simulink model "Sim_main"  (R2025a)
settings: Solver=FixedStepAuto  StartTime=0.0  StopTime=8760  FixedStep=1  RelTol=1e-3
values from neighbouring files (symbols this model uses):
  A = R * 2 * H    [LCOW_calculation.m]    (also in RUN_Simulink_POOL.m; RUN_Simulink_RandomSet.m; RUN_Simulink_SINGLE.m = 12.786871552)
  Cf = 36000    [RUN_Simulink_POOL.m]    (also in RUN_Simulink_RandomSet.m; RUN_Simulink_SINGLE.m)
  CutIn = 3    [RUN_Simulink_POOL.m]    (also in RUN_Simulink_RandomSet.m; RUN_Simulink_SINGLE.m)
  IP1 = (n/(n-1))*P1*( (P2/P1)^((n-1)/n) - 1)    (= 259255.992944)    [RUN_Simulink_POOL.m]    (also in RUN_Simulink_RandomSet.m; RUN_Simulink_SINGLE.m)
  J1 = 1.5 * As    [RUN_Simulink_POOL.m]    (also in RUN_Simulink_RandomSet.m; RUN_Simulink_SINGLE.m = 4.38)
  Limit_Tor = Tor_rq * 0.5    (= 2.3371585434)    [RUN_Simulink_POOL.m]    (also in RUN_Simulink_RandomSet.m; RUN_Simulink_SINGLE.m = 3.45899464424)
  N_PV = data.N_PV(i)    [LCOW_calculation.m]    (also in MOO_Qp_LCOW_CO2.m = optimvar("N_PV","Type","integer","LowerBound",1,"UpperBound"; RUN_Simulink_POOL.m = N_PV_values(i); RUN_Simulink_RandomSet.m = N_PV_values; RUN_Simulink_SINGLE.m = 2)
  N_ro = data.N_ro(i)    [LCOW_calculation.m]    (also in MOO_Qp_LCOW_CO2.m = optimvar("N_ro","Type","integer","LowerBound",2,"UpperBound"; RUN_Simulink_POOL.m = N_ro_values(i); RUN_Simulink_RandomSet.m = N_ro_values; RUN_Simulink_SINGLE.m = 6)
  Nt = data.Nt(i)    [LCOW_calculation.m]    (also in MOO_Qp_LCOW_CO2.m = optimvar("Nt","Type","integer","LowerBound",10,"UpperBound",; RUN_Simulink_POOL.m = Nt_values(i); RUN_Simulink_RandomSet.m = Nt_values; RUN_Simulink_SINGLE.m = 58)
  P2 = 800000    [RUN_Simulink_POOL.m]    (also in RUN_Simulink_RandomSet.m; RUN_Simulink_SINGLE.m)
  R = 0.515 * As    [LCOW_calculation.m]    (also in RUN_Simulink_POOL.m; RUN_Simulink_RandomSet.m; RUN_Simulink_SINGLE.m = 1.5038)
  Tor_rq = IP1 * Va * 10 / (17 * pi)    (= 4.67431708681)    [RUN_Simulink_POOL.m]    (also in RUN_Simulink_RandomSet.m; RUN_Simulink_SINGLE.m = 6.91798928848)
  TR = data.TR(i)    [LCOW_calculation.m]    (also in MOO_Qp_LCOW_CO2.m = optimvar("TR","LowerBound",3,"UpperBound",10); RUN_Simulink_POOL.m = TR_values(i); RUN_Simulink_RandomSet.m = TR_values; RUN_Simulink_SINGLE.m = 9.36)
  Va = e_vol * Vs    (= 9.6291546017e-05)    [RUN_Simulink_POOL.m]    (also in RUN_Simulink_RandomSet.m; RUN_Simulink_SINGLE.m = 0.000142511488105)
  Vf1 = ((P1+Pa)*T2/(T1*(P2+Pa)))*1000    (= 339.891157105)    [RUN_Simulink_POOL.m]    (also in RUN_Simulink_RandomSet.m; RUN_Simulink_SINGLE.m)
  Vt = 2000    [RUN_Simulink_POOL.m]    (also in RUN_Simulink_RandomSet.m; RUN_Simulink_SINGLE.m)
undefined symbols (not defined in the file or in its folder): magnitude
libraries: statsLibrary x36, simulink x1
(part 4 of 4)

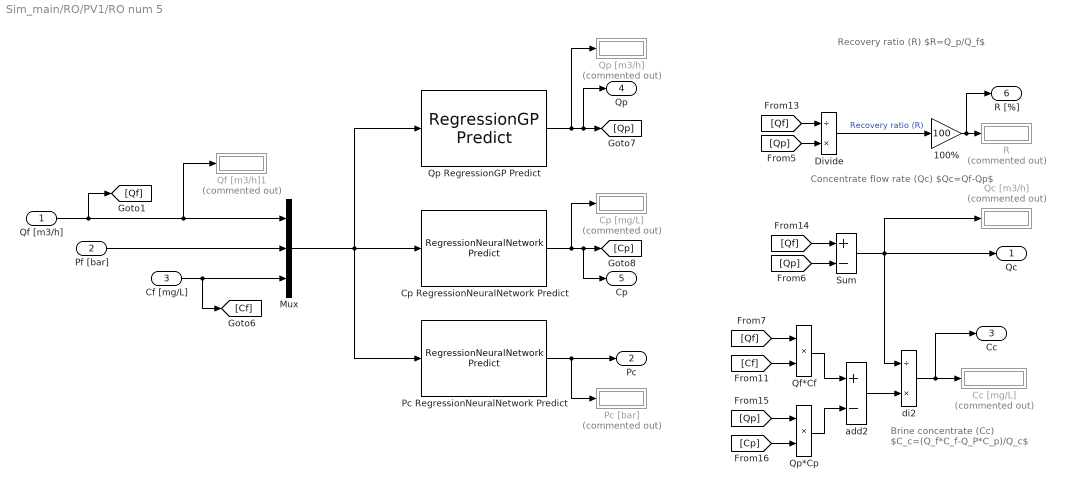
== system Sim_main/RO/PV1/RO num 5 ==
  note: Recovery ratio (R)
      | $R=Q_p/Q_f$
  note: Concentrate flow rate (Qc)
      | $Qc=Qf-Qp$
  note: Brine concentrate (Cc)
      | $C_c=(Q_f*C_f-Q_P*C_p)/Q_c$
  Qf [m3/h] : Inport
  Pf [bar] : Inport  Port=2
  Cf [mg/L] : Inport  Port=3
  100% : Gain  Gain=100
  Cc [mg/L] : Display  Commented=on
      settings: Format=bank
  Cp RegressionNeuralNetwork Predict : statsLibrary/Regression/RegressionNeuralNetwork Predict  TrainedLearner=RO_Cp.RegressionNeuralNetwork  OutMin=[]  OutMax=[]  OutputLayerOutMin=[]  OutputLayerOutMax=[]  OutputLayerAdditionOutMin=[]  OutputLayerAdditionOutMax=[]  LayerSelector=Layer 1  Layer1OutMin=[]  Layer1OutMax=[]  Layer1AdditionOutMin=[]  Layer1AdditionOutMax=[]  Layer2OutMin=[]  Layer2OutMax=[]  Layer2AdditionOutMin=[]  Layer2AdditionOutMax=[]  Layer3OutMin=[]  Layer3OutMax=[]  Layer3AdditionOutMin=[]  Layer3AdditionOutMax=[]  Layer4OutMin=[]  Layer4OutMax=[]  Layer4AdditionOutMin=[]  Layer4AdditionOutMax=[]  Layer5OutMin=[]  Layer5OutMax=[]  Layer5AdditionOutMin=[]  Layer5AdditionOutMax=[]  Layer6OutMin=[]  Layer6OutMax=[]  Layer6AdditionOutMin=[]  Layer6AdditionOutMax=[]  Layer7OutMin=[]  Layer7OutMax=[]  Layer7AdditionOutMin=[]  Layer7AdditionOutMax=[]  Layer8OutMin=[]  Layer8OutMax=[]  Layer8AdditionOutMin=[]  Layer8AdditionOutMax=[]  Layer9OutMin=[]  Layer9OutMax=[]  Layer9AdditionOutMin=[]  Layer9AdditionOutMax=[]  Layer10OutMin=[]  Layer10OutMax=[]  Layer10AdditionOutMin=[]  Layer10AdditionOutMax=[]  Layer11OutMin=[]  Layer11OutMax=[]  Layer11AdditionOutMin=[]  Layer11AdditionOutMax=[]  StandardizedInputOutMin=[]  StandardizedInputOutMax=[]  NumHiddenLayers=1
  Cp [mg/L] : Display  Commented=on
  Divide : Product  Inputs=/*
  Mux : Mux  Inputs=3
  Pc RegressionNeuralNetwork Predict : statsLibrary/Regression/RegressionNeuralNetwork Predict  TrainedLearner=RO_Pc.RegressionNeuralNetwork  OutMin=[]  OutMax=[]  OutputLayerOutMin=[]  OutputLayerOutMax=[]  OutputLayerAdditionOutMin=[]  OutputLayerAdditionOutMax=[]  LayerSelector=Layer 1  Layer1OutMin=[]  Layer1OutMax=[]  Layer1AdditionOutMin=[]  Layer1AdditionOutMax=[]  Layer2OutMin=[]  Layer2OutMax=[]  Layer2AdditionOutMin=[]  Layer2AdditionOutMax=[]  Layer3OutMin=[]  Layer3OutMax=[]  Layer3AdditionOutMin=[]  Layer3AdditionOutMax=[]  Layer4OutMin=[]  Layer4OutMax=[]  Layer4AdditionOutMin=[]  Layer4AdditionOutMax=[]  Layer5OutMin=[]  Layer5OutMax=[]  Layer5AdditionOutMin=[]  Layer5AdditionOutMax=[]  Layer6OutMin=[]  Layer6OutMax=[]  Layer6AdditionOutMin=[]  Layer6AdditionOutMax=[]  Layer7OutMin=[]  Layer7OutMax=[]  Layer7AdditionOutMin=[]  Layer7AdditionOutMax=[]  Layer8OutMin=[]  Layer8OutMax=[]  Layer8AdditionOutMin=[]  Layer8AdditionOutMax=[]  Layer9OutMin=[]  Layer9OutMax=[]  Layer9AdditionOutMin=[]  Layer9AdditionOutMax=[]  Layer10OutMin=[]  Layer10OutMax=[]  Layer10AdditionOutMin=[]  Layer10AdditionOutMax=[]  Layer11OutMin=[]  Layer11OutMax=[]  Layer11AdditionOutMin=[]  Layer11AdditionOutMax=[]  StandardizedInputOutMin=[]  StandardizedInputOutMax=[]  NumHiddenLayers=1
  Pc [bar] : Display  Commented=on
  Qc [m3/h] : Display  Commented=on
  Qf [m3/h]1 : Display  Commented=on
  Qf*Cf : Product
  Qp RegressionGP Predict : statsLibrary/Regression/RegressionGP Predict  TrainedLearner=RO_Qp.RegressionGP  ShowOutputSD=off  ShowOutputIntervals=off  Alpha=0.05  OutMin=[]  OutMax=[]  SDOutMin=[]  SDOutMax=[]  IntervalsOutMin=[]  IntervalsOutMax=[]  KernelMin=[]  KernelMax=[]  DistanceOutMin=[]  DistanceOutMax=[]  BasisOutMin=[]  BasisOutMax=[]  StandardizedInputOutMin=[]  StandardizedInputOutMax=[]  KernelParam1Min=[]  KernelParam1Max=[]  KernelParam2Min=[]  KernelParam2Max=[]  KernelParam3Min=[]  KernelParam3Max=[]  KernelParam4Min=[]  KernelParam4Max=[]  BasisParam1Min=[]  BasisParam1Max=[]  BasisParam2Min=[]  BasisParam2Max=[]  SDParam1Min=[]  SDParam1Max=[]  KernelParam5Min=[]  KernelParam5Max=[]
  Qp [m3/h] : Display  Commented=on
  Qp*Cp : Product
  R : Display  Commented=on
  Sum : Sum  Inputs=+-
  add2 : Sum  Inputs=+-
  di2 : Product  Inputs=/*
  Qc : Outport
  Pc : Outport  Port=2
  Cc : Outport  Port=3
  Qp : Outport  Port=4
  Cp : Outport  Port=5
  R [%] : Outport  Port=6
  wires:
  Cp RegressionNeuralNetwork Predict/1 -> Cp/1, [Cp], Cp [mg/L]/1
  Pc RegressionNeuralNetwork Predict/1 -> Pc/1, Pc [bar]/1
  Divide/1 -> 100%/1  "Recovery ratio (R)"
  Cf [mg/L]/1 -> Mux/3, [Cf]
  Mux/1 -> Pc RegressionNeuralNetwork Predict/1, Qp RegressionGP Predict/1, Cp RegressionNeuralNetwork Predict/1
  Pf [bar]/1 -> Mux/2
  Qf [m3/h]/1 -> [Qf], Qf [m3/h]1/1, Mux/1
  100%/1 -> R/1, R [%]/1
  Qp RegressionGP Predict/1 -> Qp/1, [Qp], Qp [m3/h]/1
  Sum/1 -> di2/1, Qc/1, Qc [m3/h]/1
  [Qf] -> Qf*Cf/1
  Qf*Cf/1 -> add2/1
  [Qp] -> Qp*Cp/1
  [Cf] -> Qf*Cf/2
  [Cp] -> Qp*Cp/2
  Qp*Cp/1 -> add2/2
  [Qf] -> Divide/1
  [Qp] -> Divide/2
  [Qf] -> Sum/1
  [Qp] -> Sum/2
  add2/1 -> di2/2
  di2/1 -> Cc/1, Cc [mg/L]/1

== system Sim_main/RO/PV1/RO num 6 ==
  note: Brine concentrate (Cc)
      | $C_c=(Q_f*C_f-Q_P*C_p)/Q_c$
  note: Concentrate flow rate (Qc)
      | $Qc=Qf-Qp$
  note: Recovery ratio (R)
      | $R=Q_p/Q_f$
  Qf [m3/h] : Inport
  Pf [bar] : Inport  Port=2
  Cf [mg/L] : Inport  Port=3
  100% : Gain  Gain=100
  Cc [mg/L] : Display  Commented=on
      settings: Format=bank
  Cp RegressionNeuralNetwork Predict : statsLibrary/Regression/RegressionNeuralNetwork Predict  TrainedLearner=RO_Cp.RegressionNeuralNetwork  OutMin=[]  OutMax=[]  OutputLayerOutMin=[]  OutputLayerOutMax=[]  OutputLayerAdditionOutMin=[]  OutputLayerAdditionOutMax=[]  LayerSelector=Layer 1  Layer1OutMin=[]  Layer1OutMax=[]  Layer1AdditionOutMin=[]  Layer1AdditionOutMax=[]  Layer2OutMin=[]  Layer2OutMax=[]  Layer2AdditionOutMin=[]  Layer2AdditionOutMax=[]  Layer3OutMin=[]  Layer3OutMax=[]  Layer3AdditionOutMin=[]  Layer3AdditionOutMax=[]  Layer4OutMin=[]  Layer4OutMax=[]  Layer4AdditionOutMin=[]  Layer4AdditionOutMax=[]  Layer5OutMin=[]  Layer5OutMax=[]  Layer5AdditionOutMin=[]  Layer5AdditionOutMax=[]  Layer6OutMin=[]  Layer6OutMax=[]  Layer6AdditionOutMin=[]  Layer6AdditionOutMax=[]  Layer7OutMin=[]  Layer7OutMax=[]  Layer7AdditionOutMin=[]  Layer7AdditionOutMax=[]  Layer8OutMin=[]  Layer8OutMax=[]  Layer8AdditionOutMin=[]  Layer8AdditionOutMax=[]  Layer9OutMin=[]  Layer9OutMax=[]  Layer9AdditionOutMin=[]  Layer9AdditionOutMax=[]  Layer10OutMin=[]  Layer10OutMax=[]  Layer10AdditionOutMin=[]  Layer10AdditionOutMax=[]  Layer11OutMin=[]  Layer11OutMax=[]  Layer11AdditionOutMin=[]  Layer11AdditionOutMax=[]  StandardizedInputOutMin=[]  StandardizedInputOutMax=[]  NumHiddenLayers=1
  Cp [mg/L] : Display  Commented=on
  Divide : Product  Inputs=/*
  Mux : Mux  Inputs=3
  Pc RegressionNeuralNetwork Predict : statsLibrary/Regression/RegressionNeuralNetwork Predict  TrainedLearner=RO_Pc.RegressionNeuralNetwork  OutMin=[]  OutMax=[]  OutputLayerOutMin=[]  OutputLayerOutMax=[]  OutputLayerAdditionOutMin=[]  OutputLayerAdditionOutMax=[]  LayerSelector=Layer 1  Layer1OutMin=[]  Layer1OutMax=[]  Layer1AdditionOutMin=[]  Layer1AdditionOutMax=[]  Layer2OutMin=[]  Layer2OutMax=[]  Layer2AdditionOutMin=[]  Layer2AdditionOutMax=[]  Layer3OutMin=[]  Layer3OutMax=[]  Layer3AdditionOutMin=[]  Layer3AdditionOutMax=[]  Layer4OutMin=[]  Layer4OutMax=[]  Layer4AdditionOutMin=[]  Layer4AdditionOutMax=[]  Layer5OutMin=[]  Layer5OutMax=[]  Layer5AdditionOutMin=[]  Layer5AdditionOutMax=[]  Layer6OutMin=[]  Layer6OutMax=[]  Layer6AdditionOutMin=[]  Layer6AdditionOutMax=[]  Layer7OutMin=[]  Layer7OutMax=[]  Layer7AdditionOutMin=[]  Layer7AdditionOutMax=[]  Layer8OutMin=[]  Layer8OutMax=[]  Layer8AdditionOutMin=[]  Layer8AdditionOutMax=[]  Layer9OutMin=[]  Layer9OutMax=[]  Layer9AdditionOutMin=[]  Layer9AdditionOutMax=[]  Layer10OutMin=[]  Layer10OutMax=[]  Layer10AdditionOutMin=[]  Layer10AdditionOutMax=[]  Layer11OutMin=[]  Layer11OutMax=[]  Layer11AdditionOutMin=[]  Layer11AdditionOutMax=[]  StandardizedInputOutMin=[]  StandardizedInputOutMax=[]  NumHiddenLayers=1
  Pc [bar] : Display  Commented=on
  Qc [m3/h] : Display  Commented=on
  Qf*Cf : Product
  Qp RegressionGP Predict : statsLibrary/Regression/RegressionGP Predict  TrainedLearner=RO_Qp.RegressionGP  ShowOutputSD=off  ShowOutputIntervals=off  Alpha=0.05  OutMin=[]  OutMax=[]  SDOutMin=[]  SDOutMax=[]  IntervalsOutMin=[]  IntervalsOutMax=[]  KernelMin=[]  KernelMax=[]  DistanceOutMin=[]  DistanceOutMax=[]  BasisOutMin=[]  BasisOutMax=[]  StandardizedInputOutMin=[]  StandardizedInputOutMax=[]  KernelParam1Min=[]  KernelParam1Max=[]  KernelParam2Min=[]  KernelParam2Max=[]  KernelParam3Min=[]  KernelParam3Max=[]  KernelParam4Min=[]  KernelParam4Max=[]  BasisParam1Min=[]  BasisParam1Max=[]  BasisParam2Min=[]  BasisParam2Max=[]  SDParam1Min=[]  SDParam1Max=[]  KernelParam5Min=[]  KernelParam5Max=[]
  Qp [m3/h] : Display  Commented=on
  Qp*Cp : Product
  R : Display  Commented=on
  Sum : Sum  Inputs=+-
  add2 : Sum  Inputs=+-
  di2 : Product  Inputs=/*
  Qc : Outport
  Pc : Outport  Port=2
  Cc : Outport  Port=3
  Qp : Outport  Port=4
  Cp : Outport  Port=5
  R [%] : Outport  Port=6
  wires:
  di2/1 -> Cc [mg/L]/1, Cc/1
  add2/1 -> di2/2
  [Qp] -> Sum/2
  [Qf] -> Sum/1
  [Qp] -> Divide/2
  [Qf] -> Divide/1
  Qp*Cp/1 -> add2/2
  [Cp] -> Qp*Cp/2
  [Cf] -> Qf*Cf/2
  [Qp] -> Qp*Cp/1
  Qf*Cf/1 -> add2/1
  [Qf] -> Qf*Cf/1
  Sum/1 -> Qc [m3/h]/1, Qc/1, di2/1
  Qp RegressionGP Predict/1 -> Qp [m3/h]/1, [Qp], Qp/1
  100%/1 -> R [%]/1, R/1
  Qf [m3/h]/1 -> Mux/1, [Qf]
  Pf [bar]/1 -> Mux/2
  Mux/1 -> Cp RegressionNeuralNetwork Predict/1, Qp RegressionGP Predict/1, Pc RegressionNeuralNetwork Predict/1
  Cf [mg/L]/1 -> [Cf], Mux/3
  Divide/1 -> 100%/1  "Recovery ratio (R)"
  Pc RegressionNeuralNetwork Predict/1 -> Pc [bar]/1, Pc/1
  Cp RegressionNeuralNetwork Predict/1 -> Cp [mg/L]/1, [Cp], Cp/1

== system Sim_main/RO/PV1/Subsystem ==
  note: product concentrate (Cp)
      | $C_3=(Q_1*C_1+Q_2*C_2)/Q_3$
  In1 : Inport
  In2 : Inport  Port=2
  In3 : Inport  Port=3
  In4 : Inport  Port=4
  Add1 : Sum
  Q1*C1 : Product
  Q2*C2 : Product
  add2 : Sum
  di2 : Product  Inputs=/*
  Out1 : Outport
  Out2 : Outport  Port=2
  wires:
  add2/1 -> di2/2
  In1/1 -> Add1/1, Q1*C1/1
  di2/1 -> Out1/1
  In3/1 -> Add1/2, Q2*C2/1
  Q1*C1/1 -> add2/1
  Q2*C2/1 -> add2/2
  Add1/1 -> di2/1, Out2/1
  In2/1 -> Q1*C1/2
  In4/1 -> Q2*C2/2

== system Sim_main/RO/PV1/Subsystem1 ==
  note: product concentrate (Cp)
      | $C_3=(Q_1*C_1+Q_2*C_2)/Q_3$
  In2 : Inport
  In3 : Inport  Port=2
  In4 : Inport  Port=3
  In1 : Inport  Port=4
  Add2 : Sum
  Q1*C1 : Product
  Q2*C2 : Product
  add2 : Sum
  di2 : Product  Inputs=/*
  Out1 : Outport
  Out2 : Outport  Port=2
  wires:
  di2/1 -> Out1/1
  add2/1 -> di2/2
  Q1*C1/1 -> add2/1
  Add2/1 -> di2/1, Out2/1
  In3/1 -> Q2*C2/1, Add2/2
  In4/1 -> Q2*C2/2
  Q2*C2/1 -> add2/2
  In2/1 -> Add2/1, Q1*C1/2
  In1/1 -> Q1*C1/1

== system Sim_main/RO/PV1/Subsystem2 ==
  note: product concentrate (Cp)
      | $C_3=(Q_1*C_1+Q_2*C_2)/Q_3$
  In2 : Inport
  In3 : Inport  Port=2
  In4 : Inport  Port=3
  In1 : Inport  Port=4
  Add2 : Sum
  Q1*C1 : Product
  Q2*C2 : Product
  add2 : Sum
  di2 : Product  Inputs=/*
  Out1 : Outport
  Out2 : Outport  Port=2
  wires:
  In1/1 -> Q1*C1/1
  In2/1 -> Q1*C1/2, Add2/1
  Q2*C2/1 -> add2/2
  In4/1 -> Q2*C2/2
  In3/1 -> Add2/2, Q2*C2/1
  Add2/1 -> Out2/1, di2/1
  Q1*C1/1 -> add2/1
  add2/1 -> di2/2
  di2/1 -> Out1/1

== system Sim_main/RO/PV1/Subsystem3 ==
  note: product concentrate (Cp)
      | $C_3=(Q_1*C_1+Q_2*C_2)/Q_3$
  In2 : Inport
  In3 : Inport  Port=2
  In4 : Inport  Port=3
  In1 : Inport  Port=4
  Add2 : Sum
  Q1*C1 : Product
  Q2*C2 : Product
  add2 : Sum
  di2 : Product  Inputs=/*
  Out1 : Outport
  wires:
  di2/1 -> Out1/1
  add2/1 -> di2/2
  Q1*C1/1 -> add2/1
  Add2/1 -> di2/1
  In3/1 -> Q2*C2/1, Add2/2
  In4/1 -> Q2*C2/2
  Q2*C2/1 -> add2/2
  In2/1 -> Add2/1, Q1*C1/2
  In1/1 -> Q1*C1/1

== system Sim_main/RO/PV1/Subsystem5 ==
  note: product concentrate (Cp)
      | $C_3=(Q_1*C_1+Q_2*C_2)/Q_3$
  In2 : Inport
  In3 : Inport  Port=2
  In4 : Inport  Port=3
  In1 : Inport  Port=4
  Add2 : Sum
  Q1*C1 : Product
  Q2*C2 : Product
  add2 : Sum
  di2 : Product  Inputs=/*
  Out1 : Outport
  Out2 : Outport  Port=2
  wires:
  In1/1 -> Q1*C1/1
  In2/1 -> Q1*C1/2, Add2/1
  Q2*C2/1 -> add2/2
  In4/1 -> Q2*C2/2
  In3/1 -> Add2/2, Q2*C2/1
  Add2/1 -> Out2/1, di2/1
  Q1*C1/1 -> add2/1
  add2/1 -> di2/2
  di2/1 -> Out1/1

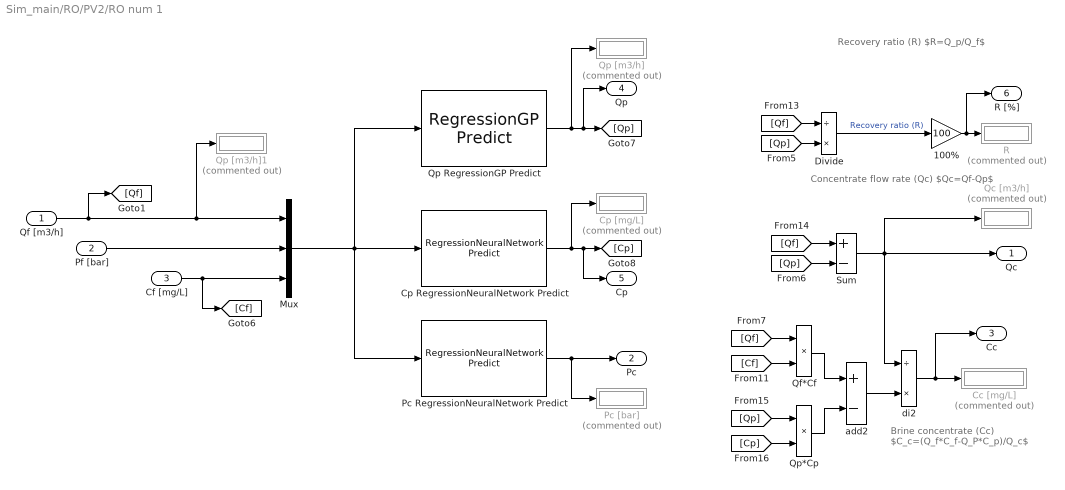
== system Sim_main/RO/PV2/RO num 1 ==
  note: Recovery ratio (R)
      | $R=Q_p/Q_f$
  note: Concentrate flow rate (Qc)
      | $Qc=Qf-Qp$
  note: Brine concentrate (Cc)
      | $C_c=(Q_f*C_f-Q_P*C_p)/Q_c$
  Qf [m3/h] : Inport
  Pf [bar] : Inport  Port=2
  Cf [mg/L] : Inport  Port=3
  100% : Gain  Gain=100
  Cc [mg/L] : Display  Commented=on
      settings: Format=bank
  Cp RegressionNeuralNetwork Predict : statsLibrary/Regression/RegressionNeuralNetwork Predict  TrainedLearner=RO_Cp.RegressionNeuralNetwork  OutMin=[]  OutMax=[]  OutputLayerOutMin=[]  OutputLayerOutMax=[]  OutputLayerAdditionOutMin=[]  OutputLayerAdditionOutMax=[]  LayerSelector=Layer 1  Layer1OutMin=[]  Layer1OutMax=[]  Layer1AdditionOutMin=[]  Layer1AdditionOutMax=[]  Layer2OutMin=[]  Layer2OutMax=[]  Layer2AdditionOutMin=[]  Layer2AdditionOutMax=[]  Layer3OutMin=[]  Layer3OutMax=[]  Layer3AdditionOutMin=[]  Layer3AdditionOutMax=[]  Layer4OutMin=[]  Layer4OutMax=[]  Layer4AdditionOutMin=[]  Layer4AdditionOutMax=[]  Layer5OutMin=[]  Layer5OutMax=[]  Layer5AdditionOutMin=[]  Layer5AdditionOutMax=[]  Layer6OutMin=[]  Layer6OutMax=[]  Layer6AdditionOutMin=[]  Layer6AdditionOutMax=[]  Layer7OutMin=[]  Layer7OutMax=[]  Layer7AdditionOutMin=[]  Layer7AdditionOutMax=[]  Layer8OutMin=[]  Layer8OutMax=[]  Layer8AdditionOutMin=[]  Layer8AdditionOutMax=[]  Layer9OutMin=[]  Layer9OutMax=[]  Layer9AdditionOutMin=[]  Layer9AdditionOutMax=[]  Layer10OutMin=[]  Layer10OutMax=[]  Layer10AdditionOutMin=[]  Layer10AdditionOutMax=[]  Layer11OutMin=[]  Layer11OutMax=[]  Layer11AdditionOutMin=[]  Layer11AdditionOutMax=[]  StandardizedInputOutMin=[]  StandardizedInputOutMax=[]  NumHiddenLayers=1
  Cp [mg/L] : Display  Commented=on
  Divide : Product  Inputs=/*
  Mux : Mux  Inputs=3
  Pc RegressionNeuralNetwork Predict : statsLibrary/Regression/RegressionNeuralNetwork Predict  TrainedLearner=RO_Pc.RegressionNeuralNetwork  OutMin=[]  OutMax=[]  OutputLayerOutMin=[]  OutputLayerOutMax=[]  OutputLayerAdditionOutMin=[]  OutputLayerAdditionOutMax=[]  LayerSelector=Layer 1  Layer1OutMin=[]  Layer1OutMax=[]  Layer1AdditionOutMin=[]  Layer1AdditionOutMax=[]  Layer2OutMin=[]  Layer2OutMax=[]  Layer2AdditionOutMin=[]  Layer2AdditionOutMax=[]  Layer3OutMin=[]  Layer3OutMax=[]  Layer3AdditionOutMin=[]  Layer3AdditionOutMax=[]  Layer4OutMin=[]  Layer4OutMax=[]  Layer4AdditionOutMin=[]  Layer4AdditionOutMax=[]  Layer5OutMin=[]  Layer5OutMax=[]  Layer5AdditionOutMin=[]  Layer5AdditionOutMax=[]  Layer6OutMin=[]  Layer6OutMax=[]  Layer6AdditionOutMin=[]  Layer6AdditionOutMax=[]  Layer7OutMin=[]  Layer7OutMax=[]  Layer7AdditionOutMin=[]  Layer7AdditionOutMax=[]  Layer8OutMin=[]  Layer8OutMax=[]  Layer8AdditionOutMin=[]  Layer8AdditionOutMax=[]  Layer9OutMin=[]  Layer9OutMax=[]  Layer9AdditionOutMin=[]  Layer9AdditionOutMax=[]  Layer10OutMin=[]  Layer10OutMax=[]  Layer10AdditionOutMin=[]  Layer10AdditionOutMax=[]  Layer11OutMin=[]  Layer11OutMax=[]  Layer11AdditionOutMin=[]  Layer11AdditionOutMax=[]  StandardizedInputOutMin=[]  StandardizedInputOutMax=[]  NumHiddenLayers=1
  Pc [bar] : Display  Commented=on
  Qc [m3/h] : Display  Commented=on
  Qf*Cf : Product
  Qp RegressionGP Predict : statsLibrary/Regression/RegressionGP Predict  TrainedLearner=RO_Qp.RegressionGP  ShowOutputSD=off  ShowOutputIntervals=off  Alpha=0.05  OutMin=[]  OutMax=[]  SDOutMin=[]  SDOutMax=[]  IntervalsOutMin=[]  IntervalsOutMax=[]  KernelMin=[]  KernelMax=[]  DistanceOutMin=[]  DistanceOutMax=[]  BasisOutMin=[]  BasisOutMax=[]  StandardizedInputOutMin=[]  StandardizedInputOutMax=[]  KernelParam1Min=[]  KernelParam1Max=[]  KernelParam2Min=[]  KernelParam2Max=[]  KernelParam3Min=[]  KernelParam3Max=[]  KernelParam4Min=[]  KernelParam4Max=[]  BasisParam1Min=[]  BasisParam1Max=[]  BasisParam2Min=[]  BasisParam2Max=[]  SDParam1Min=[]  SDParam1Max=[]  KernelParam5Min=[]  KernelParam5Max=[]
  Qp [m3/h] : Display  Commented=on
  Qp [m3/h]1 : Display  Commented=on
  Qp*Cp : Product
  R : Display  Commented=on
  Sum : Sum  Inputs=+-
  add2 : Sum  Inputs=+-
  di2 : Product  Inputs=/*
  Qc : Outport
  Pc : Outport  Port=2
  Cc : Outport  Port=3
  Qp : Outport  Port=4
  Cp : Outport  Port=5
  R [%] : Outport  Port=6
  wires:
  Cp RegressionNeuralNetwork Predict/1 -> Cp/1, [Cp], Cp [mg/L]/1
  Pc RegressionNeuralNetwork Predict/1 -> Pc/1, Pc [bar]/1
  Divide/1 -> 100%/1  "Recovery ratio (R)"
  Cf [mg/L]/1 -> Mux/3, [Cf]
  Mux/1 -> Pc RegressionNeuralNetwork Predict/1, Qp RegressionGP Predict/1, Cp RegressionNeuralNetwork Predict/1
  Pf [bar]/1 -> Mux/2
  100%/1 -> R/1, R [%]/1
  Qp RegressionGP Predict/1 -> Qp/1, [Qp], Qp [m3/h]/1
  Sum/1 -> di2/1, Qc/1, Qc [m3/h]/1
  [Qf] -> Qf*Cf/1
  Qf*Cf/1 -> add2/1
  [Qp] -> Qp*Cp/1
  [Cf] -> Qf*Cf/2
  [Cp] -> Qp*Cp/2
  Qp*Cp/1 -> add2/2
  [Qf] -> Divide/1
  [Qp] -> Divide/2
  [Qf] -> Sum/1
  [Qp] -> Sum/2
  add2/1 -> di2/2
  di2/1 -> Cc/1, Cc [mg/L]/1
  Qf [m3/h]/1 -> [Qf], Mux/1, Qp [m3/h]1/1

== system Sim_main/RO/PV2/RO num 2 ==
  note: Brine concentrate (Cc)
      | $C_c=(Q_f*C_f-Q_P*C_p)/Q_c$
  note: Concentrate flow rate (Qc)
      | $Qc=Qf-Qp$
  note: Recovery ratio (R)
      | $R=Q_p/Q_f$
  Qf [m3/h] : Inport
  Pf [bar] : Inport  Port=2
  Cf [mg/L] : Inport  Port=3
  100% : Gain  Gain=100
  Cc [mg/L] : Display  Commented=on
      settings: Format=bank
  Cp RegressionNeuralNetwork Predict : statsLibrary/Regression/RegressionNeuralNetwork Predict  TrainedLearner=RO_Cp.RegressionNeuralNetwork  OutMin=[]  OutMax=[]  OutputLayerOutMin=[]  OutputLayerOutMax=[]  OutputLayerAdditionOutMin=[]  OutputLayerAdditionOutMax=[]  LayerSelector=Layer 1  Layer1OutMin=[]  Layer1OutMax=[]  Layer1AdditionOutMin=[]  Layer1AdditionOutMax=[]  Layer2OutMin=[]  Layer2OutMax=[]  Layer2AdditionOutMin=[]  Layer2AdditionOutMax=[]  Layer3OutMin=[]  Layer3OutMax=[]  Layer3AdditionOutMin=[]  Layer3AdditionOutMax=[]  Layer4OutMin=[]  Layer4OutMax=[]  Layer4AdditionOutMin=[]  Layer4AdditionOutMax=[]  Layer5OutMin=[]  Layer5OutMax=[]  Layer5AdditionOutMin=[]  Layer5AdditionOutMax=[]  Layer6OutMin=[]  Layer6OutMax=[]  Layer6AdditionOutMin=[]  Layer6AdditionOutMax=[]  Layer7OutMin=[]  Layer7OutMax=[]  Layer7AdditionOutMin=[]  Layer7AdditionOutMax=[]  Layer8OutMin=[]  Layer8OutMax=[]  Layer8AdditionOutMin=[]  Layer8AdditionOutMax=[]  Layer9OutMin=[]  Layer9OutMax=[]  Layer9AdditionOutMin=[]  Layer9AdditionOutMax=[]  Layer10OutMin=[]  Layer10OutMax=[]  Layer10AdditionOutMin=[]  Layer10AdditionOutMax=[]  Layer11OutMin=[]  Layer11OutMax=[]  Layer11AdditionOutMin=[]  Layer11AdditionOutMax=[]  StandardizedInputOutMin=[]  StandardizedInputOutMax=[]  NumHiddenLayers=1
  Cp [mg/L] : Display  Commented=on
  Divide : Product  Inputs=/*
  Mux : Mux  Inputs=3
  Pc RegressionNeuralNetwork Predict : statsLibrary/Regression/RegressionNeuralNetwork Predict  TrainedLearner=RO_Pc.RegressionNeuralNetwork  OutMin=[]  OutMax=[]  OutputLayerOutMin=[]  OutputLayerOutMax=[]  OutputLayerAdditionOutMin=[]  OutputLayerAdditionOutMax=[]  LayerSelector=Layer 1  Layer1OutMin=[]  Layer1OutMax=[]  Layer1AdditionOutMin=[]  Layer1AdditionOutMax=[]  Layer2OutMin=[]  Layer2OutMax=[]  Layer2AdditionOutMin=[]  Layer2AdditionOutMax=[]  Layer3OutMin=[]  Layer3OutMax=[]  Layer3AdditionOutMin=[]  Layer3AdditionOutMax=[]  Layer4OutMin=[]  Layer4OutMax=[]  Layer4AdditionOutMin=[]  Layer4AdditionOutMax=[]  Layer5OutMin=[]  Layer5OutMax=[]  Layer5AdditionOutMin=[]  Layer5AdditionOutMax=[]  Layer6OutMin=[]  Layer6OutMax=[]  Layer6AdditionOutMin=[]  Layer6AdditionOutMax=[]  Layer7OutMin=[]  Layer7OutMax=[]  Layer7AdditionOutMin=[]  Layer7AdditionOutMax=[]  Layer8OutMin=[]  Layer8OutMax=[]  Layer8AdditionOutMin=[]  Layer8AdditionOutMax=[]  Layer9OutMin=[]  Layer9OutMax=[]  Layer9AdditionOutMin=[]  Layer9AdditionOutMax=[]  Layer10OutMin=[]  Layer10OutMax=[]  Layer10AdditionOutMin=[]  Layer10AdditionOutMax=[]  Layer11OutMin=[]  Layer11OutMax=[]  Layer11AdditionOutMin=[]  Layer11AdditionOutMax=[]  StandardizedInputOutMin=[]  StandardizedInputOutMax=[]  NumHiddenLayers=1
  Pc [bar] : Display  Commented=on
  Qc [m3/h] : Display  Commented=on
  Qf*Cf : Product
  Qp RegressionGP Predict : statsLibrary/Regression/RegressionGP Predict  TrainedLearner=RO_Qp.RegressionGP  ShowOutputSD=off  ShowOutputIntervals=off  Alpha=0.05  OutMin=[]  OutMax=[]  SDOutMin=[]  SDOutMax=[]  IntervalsOutMin=[]  IntervalsOutMax=[]  KernelMin=[]  KernelMax=[]  DistanceOutMin=[]  DistanceOutMax=[]  BasisOutMin=[]  BasisOutMax=[]  StandardizedInputOutMin=[]  StandardizedInputOutMax=[]  KernelParam1Min=[]  KernelParam1Max=[]  KernelParam2Min=[]  KernelParam2Max=[]  KernelParam3Min=[]  KernelParam3Max=[]  KernelParam4Min=[]  KernelParam4Max=[]  BasisParam1Min=[]  BasisParam1Max=[]  BasisParam2Min=[]  BasisParam2Max=[]  SDParam1Min=[]  SDParam1Max=[]  KernelParam5Min=[]  KernelParam5Max=[]
  Qp [m3/h] : Display  Commented=on
  Qp*Cp : Product
  R : Display  Commented=on
  Sum : Sum  Inputs=+-
  add2 : Sum  Inputs=+-
  di2 : Product  Inputs=/*
  Qc : Outport
  Pc : Outport  Port=2
  Cc : Outport  Port=3
  Qp : Outport  Port=4
  Cp : Outport  Port=5
  R [%] : Outport  Port=6
  wires:
  di2/1 -> Cc [mg/L]/1, Cc/1
  add2/1 -> di2/2
  [Qp] -> Sum/2
  [Qf] -> Sum/1
  [Qp] -> Divide/2
  [Qf] -> Divide/1
  Qp*Cp/1 -> add2/2
  [Cp] -> Qp*Cp/2
  [Cf] -> Qf*Cf/2
  [Qp] -> Qp*Cp/1
  Qf*Cf/1 -> add2/1
  [Qf] -> Qf*Cf/1
  Sum/1 -> Qc [m3/h]/1, Qc/1, di2/1
  Qp RegressionGP Predict/1 -> Qp [m3/h]/1, [Qp], Qp/1
  100%/1 -> R [%]/1, R/1
  Qf [m3/h]/1 -> Mux/1, [Qf]
  Pf [bar]/1 -> Mux/2
  Mux/1 -> Cp RegressionNeuralNetwork Predict/1, Qp RegressionGP Predict/1, Pc RegressionNeuralNetwork Predict/1
  Cf [mg/L]/1 -> [Cf], Mux/3
  Divide/1 -> 100%/1  "Recovery ratio (R)"
  Pc RegressionNeuralNetwork Predict/1 -> Pc [bar]/1, Pc/1
  Cp RegressionNeuralNetwork Predict/1 -> Cp [mg/L]/1, [Cp], Cp/1

== system Sim_main/RO/PV2/RO num 3 ==
  note: Recovery ratio (R)
      | $R=Q_p/Q_f$
  note: Concentrate flow rate (Qc)
      | $Qc=Qf-Qp$
  note: Brine concentrate (Cc)
      | $C_c=(Q_f*C_f-Q_P*C_p)/Q_c$
  Qf [m3/h] : Inport
  Pf [bar] : Inport  Port=2
  Cf [mg/L] : Inport  Port=3
  100% : Gain  Gain=100
  Cc [mg/L] : Display  Commented=on
      settings: Format=bank
  Cp RegressionNeuralNetwork Predict : statsLibrary/Regression/RegressionNeuralNetwork Predict  TrainedLearner=RO_Cp.RegressionNeuralNetwork  OutMin=[]  OutMax=[]  OutputLayerOutMin=[]  OutputLayerOutMax=[]  OutputLayerAdditionOutMin=[]  OutputLayerAdditionOutMax=[]  LayerSelector=Layer 1  Layer1OutMin=[]  Layer1OutMax=[]  Layer1AdditionOutMin=[]  Layer1AdditionOutMax=[]  Layer2OutMin=[]  Layer2OutMax=[]  Layer2AdditionOutMin=[]  Layer2AdditionOutMax=[]  Layer3OutMin=[]  Layer3OutMax=[]  Layer3AdditionOutMin=[]  Layer3AdditionOutMax=[]  Layer4OutMin=[]  Layer4OutMax=[]  Layer4AdditionOutMin=[]  Layer4AdditionOutMax=[]  Layer5OutMin=[]  Layer5OutMax=[]  Layer5AdditionOutMin=[]  Layer5AdditionOutMax=[]  Layer6OutMin=[]  Layer6OutMax=[]  Layer6AdditionOutMin=[]  Layer6AdditionOutMax=[]  Layer7OutMin=[]  Layer7OutMax=[]  Layer7AdditionOutMin=[]  Layer7AdditionOutMax=[]  Layer8OutMin=[]  Layer8OutMax=[]  Layer8AdditionOutMin=[]  Layer8AdditionOutMax=[]  Layer9OutMin=[]  Layer9OutMax=[]  Layer9AdditionOutMin=[]  Layer9AdditionOutMax=[]  Layer10OutMin=[]  Layer10OutMax=[]  Layer10AdditionOutMin=[]  Layer10AdditionOutMax=[]  Layer11OutMin=[]  Layer11OutMax=[]  Layer11AdditionOutMin=[]  Layer11AdditionOutMax=[]  StandardizedInputOutMin=[]  StandardizedInputOutMax=[]  NumHiddenLayers=1
  Cp [mg/L] : Display  Commented=on
  Divide : Product  Inputs=/*
  Mux : Mux  Inputs=3
  Pc RegressionNeuralNetwork Predict : statsLibrary/Regression/RegressionNeuralNetwork Predict  TrainedLearner=RO_Pc.RegressionNeuralNetwork  OutMin=[]  OutMax=[]  OutputLayerOutMin=[]  OutputLayerOutMax=[]  OutputLayerAdditionOutMin=[]  OutputLayerAdditionOutMax=[]  LayerSelector=Layer 1  Layer1OutMin=[]  Layer1OutMax=[]  Layer1AdditionOutMin=[]  Layer1AdditionOutMax=[]  Layer2OutMin=[]  Layer2OutMax=[]  Layer2AdditionOutMin=[]  Layer2AdditionOutMax=[]  Layer3OutMin=[]  Layer3OutMax=[]  Layer3AdditionOutMin=[]  Layer3AdditionOutMax=[]  Layer4OutMin=[]  Layer4OutMax=[]  Layer4AdditionOutMin=[]  Layer4AdditionOutMax=[]  Layer5OutMin=[]  Layer5OutMax=[]  Layer5AdditionOutMin=[]  Layer5AdditionOutMax=[]  Layer6OutMin=[]  Layer6OutMax=[]  Layer6AdditionOutMin=[]  Layer6AdditionOutMax=[]  Layer7OutMin=[]  Layer7OutMax=[]  Layer7AdditionOutMin=[]  Layer7AdditionOutMax=[]  Layer8OutMin=[]  Layer8OutMax=[]  Layer8AdditionOutMin=[]  Layer8AdditionOutMax=[]  Layer9OutMin=[]  Layer9OutMax=[]  Layer9AdditionOutMin=[]  Layer9AdditionOutMax=[]  Layer10OutMin=[]  Layer10OutMax=[]  Layer10AdditionOutMin=[]  Layer10AdditionOutMax=[]  Layer11OutMin=[]  Layer11OutMax=[]  Layer11AdditionOutMin=[]  Layer11AdditionOutMax=[]  StandardizedInputOutMin=[]  StandardizedInputOutMax=[]  NumHiddenLayers=1
  Pc [bar] : Display  Commented=on
  Qc [m3/h] : Display  Commented=on
  Qf*Cf : Product
  Qp RegressionGP Predict : statsLibrary/Regression/RegressionGP Predict  TrainedLearner=RO_Qp.RegressionGP  ShowOutputSD=off  ShowOutputIntervals=off  Alpha=0.05  OutMin=[]  OutMax=[]  SDOutMin=[]  SDOutMax=[]  IntervalsOutMin=[]  IntervalsOutMax=[]  KernelMin=[]  KernelMax=[]  DistanceOutMin=[]  DistanceOutMax=[]  BasisOutMin=[]  BasisOutMax=[]  StandardizedInputOutMin=[]  StandardizedInputOutMax=[]  KernelParam1Min=[]  KernelParam1Max=[]  KernelParam2Min=[]  KernelParam2Max=[]  KernelParam3Min=[]  KernelParam3Max=[]  KernelParam4Min=[]  KernelParam4Max=[]  BasisParam1Min=[]  BasisParam1Max=[]  BasisParam2Min=[]  BasisParam2Max=[]  SDParam1Min=[]  SDParam1Max=[]  KernelParam5Min=[]  KernelParam5Max=[]
  Qp [m3/h] : Display  Commented=on
  Qp*Cp : Product
  R : Display  Commented=on
  Sum : Sum  Inputs=+-
  add2 : Sum  Inputs=+-
  di2 : Product  Inputs=/*
  Qc : Outport
  Pc : Outport  Port=2
  Cc : Outport  Port=3
  Qp : Outport  Port=4
  Cp : Outport  Port=5
  R [%] : Outport  Port=6
  wires:
  Cp RegressionNeuralNetwork Predict/1 -> Cp/1, [Cp], Cp [mg/L]/1
  Pc RegressionNeuralNetwork Predict/1 -> Pc/1, Pc [bar]/1
  Divide/1 -> 100%/1  "Recovery ratio (R)"
  Cf [mg/L]/1 -> Mux/3, [Cf]
  Mux/1 -> Pc RegressionNeuralNetwork Predict/1, Qp RegressionGP Predict/1, Cp RegressionNeuralNetwork Predict/1
  Pf [bar]/1 -> Mux/2
  Qf [m3/h]/1 -> [Qf], Mux/1
  100%/1 -> R/1, R [%]/1
  Qp RegressionGP Predict/1 -> Qp/1, [Qp], Qp [m3/h]/1
  Sum/1 -> di2/1, Qc/1, Qc [m3/h]/1
  [Qf] -> Qf*Cf/1
  Qf*Cf/1 -> add2/1
  [Qp] -> Qp*Cp/1
  [Cf] -> Qf*Cf/2
  [Cp] -> Qp*Cp/2
  Qp*Cp/1 -> add2/2
  [Qf] -> Divide/1
  [Qp] -> Divide/2
  [Qf] -> Sum/1
  [Qp] -> Sum/2
  add2/1 -> di2/2
  di2/1 -> Cc/1, Cc [mg/L]/1

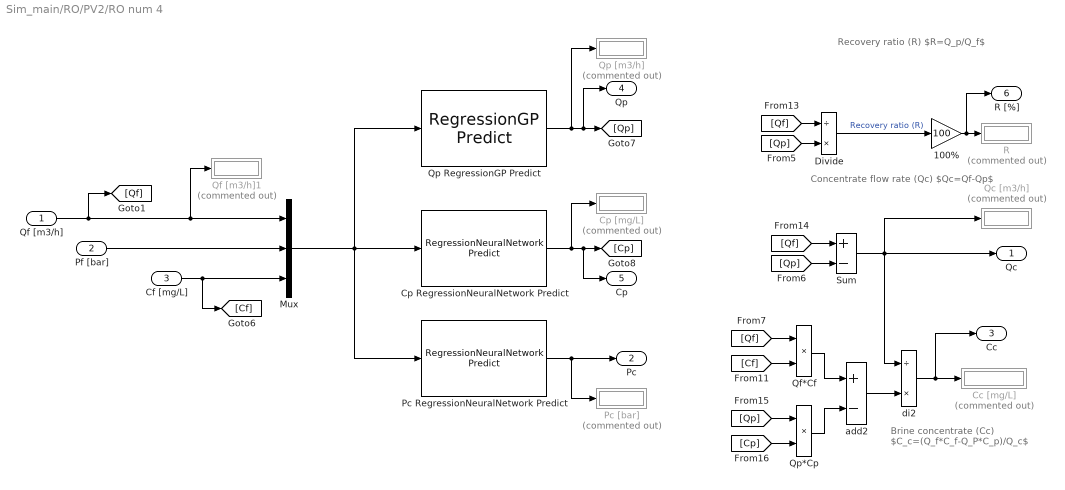
== system Sim_main/RO/PV2/RO num 4 ==
  note: Brine concentrate (Cc)
      | $C_c=(Q_f*C_f-Q_P*C_p)/Q_c$
  note: Concentrate flow rate (Qc)
      | $Qc=Qf-Qp$
  note: Recovery ratio (R)
      | $R=Q_p/Q_f$
  Qf [m3/h] : Inport
  Pf [bar] : Inport  Port=2
  Cf [mg/L] : Inport  Port=3
  100% : Gain  Gain=100
  Cc [mg/L] : Display  Commented=on
      settings: Format=bank
  Cp RegressionNeuralNetwork Predict : statsLibrary/Regression/RegressionNeuralNetwork Predict  TrainedLearner=RO_Cp.RegressionNeuralNetwork  OutMin=[]  OutMax=[]  OutputLayerOutMin=[]  OutputLayerOutMax=[]  OutputLayerAdditionOutMin=[]  OutputLayerAdditionOutMax=[]  LayerSelector=Layer 1  Layer1OutMin=[]  Layer1OutMax=[]  Layer1AdditionOutMin=[]  Layer1AdditionOutMax=[]  Layer2OutMin=[]  Layer2OutMax=[]  Layer2AdditionOutMin=[]  Layer2AdditionOutMax=[]  Layer3OutMin=[]  Layer3OutMax=[]  Layer3AdditionOutMin=[]  Layer3AdditionOutMax=[]  Layer4OutMin=[]  Layer4OutMax=[]  Layer4AdditionOutMin=[]  Layer4AdditionOutMax=[]  Layer5OutMin=[]  Layer5OutMax=[]  Layer5AdditionOutMin=[]  Layer5AdditionOutMax=[]  Layer6OutMin=[]  Layer6OutMax=[]  Layer6AdditionOutMin=[]  Layer6AdditionOutMax=[]  Layer7OutMin=[]  Layer7OutMax=[]  Layer7AdditionOutMin=[]  Layer7AdditionOutMax=[]  Layer8OutMin=[]  Layer8OutMax=[]  Layer8AdditionOutMin=[]  Layer8AdditionOutMax=[]  Layer9OutMin=[]  Layer9OutMax=[]  Layer9AdditionOutMin=[]  Layer9AdditionOutMax=[]  Layer10OutMin=[]  Layer10OutMax=[]  Layer10AdditionOutMin=[]  Layer10AdditionOutMax=[]  Layer11OutMin=[]  Layer11OutMax=[]  Layer11AdditionOutMin=[]  Layer11AdditionOutMax=[]  StandardizedInputOutMin=[]  StandardizedInputOutMax=[]  NumHiddenLayers=1
  Cp [mg/L] : Display  Commented=on
  Divide : Product  Inputs=/*
  Mux : Mux  Inputs=3
  Pc RegressionNeuralNetwork Predict : statsLibrary/Regression/RegressionNeuralNetwork Predict  TrainedLearner=RO_Pc.RegressionNeuralNetwork  OutMin=[]  OutMax=[]  OutputLayerOutMin=[]  OutputLayerOutMax=[]  OutputLayerAdditionOutMin=[]  OutputLayerAdditionOutMax=[]  LayerSelector=Layer 1  Layer1OutMin=[]  Layer1OutMax=[]  Layer1AdditionOutMin=[]  Layer1AdditionOutMax=[]  Layer2OutMin=[]  Layer2OutMax=[]  Layer2AdditionOutMin=[]  Layer2AdditionOutMax=[]  Layer3OutMin=[]  Layer3OutMax=[]  Layer3AdditionOutMin=[]  Layer3AdditionOutMax=[]  Layer4OutMin=[]  Layer4OutMax=[]  Layer4AdditionOutMin=[]  Layer4AdditionOutMax=[]  Layer5OutMin=[]  Layer5OutMax=[]  Layer5AdditionOutMin=[]  Layer5AdditionOutMax=[]  Layer6OutMin=[]  Layer6OutMax=[]  Layer6AdditionOutMin=[]  Layer6AdditionOutMax=[]  Layer7OutMin=[]  Layer7OutMax=[]  Layer7AdditionOutMin=[]  Layer7AdditionOutMax=[]  Layer8OutMin=[]  Layer8OutMax=[]  Layer8AdditionOutMin=[]  Layer8AdditionOutMax=[]  Layer9OutMin=[]  Layer9OutMax=[]  Layer9AdditionOutMin=[]  Layer9AdditionOutMax=[]  Layer10OutMin=[]  Layer10OutMax=[]  Layer10AdditionOutMin=[]  Layer10AdditionOutMax=[]  Layer11OutMin=[]  Layer11OutMax=[]  Layer11AdditionOutMin=[]  Layer11AdditionOutMax=[]  StandardizedInputOutMin=[]  StandardizedInputOutMax=[]  NumHiddenLayers=1
  Pc [bar] : Display  Commented=on
  Qc [m3/h] : Display  Commented=on
  Qf [m3/h]1 : Display  Commented=on
  Qf*Cf : Product
  Qp RegressionGP Predict : statsLibrary/Regression/RegressionGP Predict  TrainedLearner=RO_Qp.RegressionGP  ShowOutputSD=off  ShowOutputIntervals=off  Alpha=0.05  OutMin=[]  OutMax=[]  SDOutMin=[]  SDOutMax=[]  IntervalsOutMin=[]  IntervalsOutMax=[]  KernelMin=[]  KernelMax=[]  DistanceOutMin=[]  DistanceOutMax=[]  BasisOutMin=[]  BasisOutMax=[]  StandardizedInputOutMin=[]  StandardizedInputOutMax=[]  KernelParam1Min=[]  KernelParam1Max=[]  KernelParam2Min=[]  KernelParam2Max=[]  KernelParam3Min=[]  KernelParam3Max=[]  KernelParam4Min=[]  KernelParam4Max=[]  BasisParam1Min=[]  BasisParam1Max=[]  BasisParam2Min=[]  BasisParam2Max=[]  SDParam1Min=[]  SDParam1Max=[]  KernelParam5Min=[]  KernelParam5Max=[]
  Qp [m3/h] : Display  Commented=on
  Qp*Cp : Product
  R : Display  Commented=on
  Sum : Sum  Inputs=+-
  add2 : Sum  Inputs=+-
  di2 : Product  Inputs=/*
  Qc : Outport
  Pc : Outport  Port=2
  Cc : Outport  Port=3
  Qp : Outport  Port=4
  Cp : Outport  Port=5
  R [%] : Outport  Port=6
  wires:
  di2/1 -> Cc [mg/L]/1, Cc/1
  add2/1 -> di2/2
  [Qp] -> Sum/2
  [Qf] -> Sum/1
  [Qp] -> Divide/2
  [Qf] -> Divide/1
  Qp*Cp/1 -> add2/2
  [Cp] -> Qp*Cp/2
  [Cf] -> Qf*Cf/2
  [Qp] -> Qp*Cp/1
  Qf*Cf/1 -> add2/1
  [Qf] -> Qf*Cf/1
  Sum/1 -> Qc [m3/h]/1, Qc/1, di2/1
  Qp RegressionGP Predict/1 -> Qp [m3/h]/1, [Qp], Qp/1
  100%/1 -> R [%]/1, R/1
  Qf [m3/h]/1 -> Qf [m3/h]1/1, Mux/1, [Qf]
  Pf [bar]/1 -> Mux/2
  Mux/1 -> Cp RegressionNeuralNetwork Predict/1, Qp RegressionGP Predict/1, Pc RegressionNeuralNetwork Predict/1
  Cf [mg/L]/1 -> [Cf], Mux/3
  Divide/1 -> 100%/1  "Recovery ratio (R)"
  Pc RegressionNeuralNetwork Predict/1 -> Pc [bar]/1, Pc/1
  Cp RegressionNeuralNetwork Predict/1 -> Cp [mg/L]/1, [Cp], Cp/1

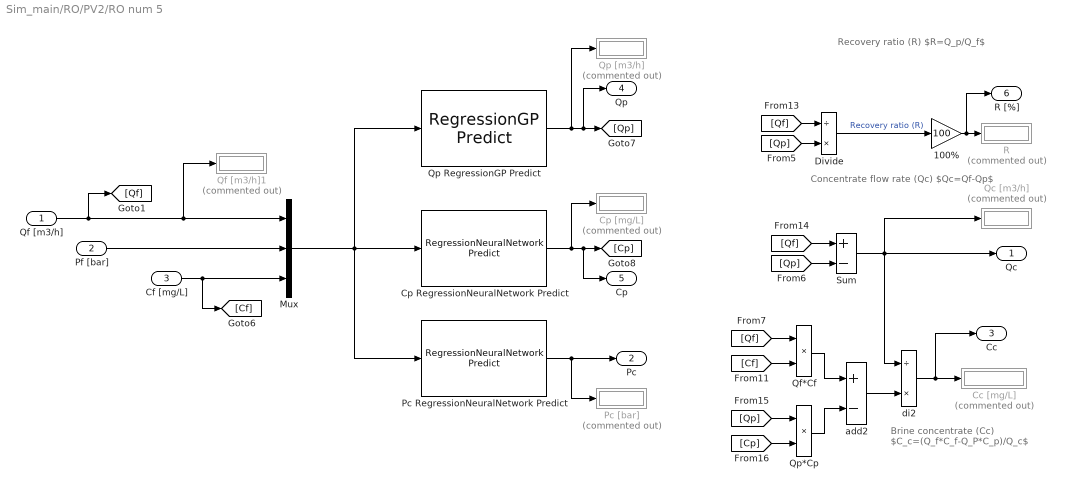
== system Sim_main/RO/PV2/RO num 5 ==
  note: Recovery ratio (R)
      | $R=Q_p/Q_f$
  note: Concentrate flow rate (Qc)
      | $Qc=Qf-Qp$
  note: Brine concentrate (Cc)
      | $C_c=(Q_f*C_f-Q_P*C_p)/Q_c$
  Qf [m3/h] : Inport
  Pf [bar] : Inport  Port=2
  Cf [mg/L] : Inport  Port=3
  100% : Gain  Gain=100
  Cc [mg/L] : Display  Commented=on
      settings: Format=bank
  Cp RegressionNeuralNetwork Predict : statsLibrary/Regression/RegressionNeuralNetwork Predict  TrainedLearner=RO_Cp.RegressionNeuralNetwork  OutMin=[]  OutMax=[]  OutputLayerOutMin=[]  OutputLayerOutMax=[]  OutputLayerAdditionOutMin=[]  OutputLayerAdditionOutMax=[]  LayerSelector=Layer 1  Layer1OutMin=[]  Layer1OutMax=[]  Layer1AdditionOutMin=[]  Layer1AdditionOutMax=[]  Layer2OutMin=[]  Layer2OutMax=[]  Layer2AdditionOutMin=[]  Layer2AdditionOutMax=[]  Layer3OutMin=[]  Layer3OutMax=[]  Layer3AdditionOutMin=[]  Layer3AdditionOutMax=[]  Layer4OutMin=[]  Layer4OutMax=[]  Layer4AdditionOutMin=[]  Layer4AdditionOutMax=[]  Layer5OutMin=[]  Layer5OutMax=[]  Layer5AdditionOutMin=[]  Layer5AdditionOutMax=[]  Layer6OutMin=[]  Layer6OutMax=[]  Layer6AdditionOutMin=[]  Layer6AdditionOutMax=[]  Layer7OutMin=[]  Layer7OutMax=[]  Layer7AdditionOutMin=[]  Layer7AdditionOutMax=[]  Layer8OutMin=[]  Layer8OutMax=[]  Layer8AdditionOutMin=[]  Layer8AdditionOutMax=[]  Layer9OutMin=[]  Layer9OutMax=[]  Layer9AdditionOutMin=[]  Layer9AdditionOutMax=[]  Layer10OutMin=[]  Layer10OutMax=[]  Layer10AdditionOutMin=[]  Layer10AdditionOutMax=[]  Layer11OutMin=[]  Layer11OutMax=[]  Layer11AdditionOutMin=[]  Layer11AdditionOutMax=[]  StandardizedInputOutMin=[]  StandardizedInputOutMax=[]  NumHiddenLayers=1
  Cp [mg/L] : Display  Commented=on
  Divide : Product  Inputs=/*
  Mux : Mux  Inputs=3
  Pc RegressionNeuralNetwork Predict : statsLibrary/Regression/RegressionNeuralNetwork Predict  TrainedLearner=RO_Pc.RegressionNeuralNetwork  OutMin=[]  OutMax=[]  OutputLayerOutMin=[]  OutputLayerOutMax=[]  OutputLayerAdditionOutMin=[]  OutputLayerAdditionOutMax=[]  LayerSelector=Layer 1  Layer1OutMin=[]  Layer1OutMax=[]  Layer1AdditionOutMin=[]  Layer1AdditionOutMax=[]  Layer2OutMin=[]  Layer2OutMax=[]  Layer2AdditionOutMin=[]  Layer2AdditionOutMax=[]  Layer3OutMin=[]  Layer3OutMax=[]  Layer3AdditionOutMin=[]  Layer3AdditionOutMax=[]  Layer4OutMin=[]  Layer4OutMax=[]  Layer4AdditionOutMin=[]  Layer4AdditionOutMax=[]  Layer5OutMin=[]  Layer5OutMax=[]  Layer5AdditionOutMin=[]  Layer5AdditionOutMax=[]  Layer6OutMin=[]  Layer6OutMax=[]  Layer6AdditionOutMin=[]  Layer6AdditionOutMax=[]  Layer7OutMin=[]  Layer7OutMax=[]  Layer7AdditionOutMin=[]  Layer7AdditionOutMax=[]  Layer8OutMin=[]  Layer8OutMax=[]  Layer8AdditionOutMin=[]  Layer8AdditionOutMax=[]  Layer9OutMin=[]  Layer9OutMax=[]  Layer9AdditionOutMin=[]  Layer9AdditionOutMax=[]  Layer10OutMin=[]  Layer10OutMax=[]  Layer10AdditionOutMin=[]  Layer10AdditionOutMax=[]  Layer11OutMin=[]  Layer11OutMax=[]  Layer11AdditionOutMin=[]  Layer11AdditionOutMax=[]  StandardizedInputOutMin=[]  StandardizedInputOutMax=[]  NumHiddenLayers=1
  Pc [bar] : Display  Commented=on
  Qc [m3/h] : Display  Commented=on
  Qf [m3/h]1 : Display  Commented=on
  Qf*Cf : Product
  Qp RegressionGP Predict : statsLibrary/Regression/RegressionGP Predict  TrainedLearner=RO_Qp.RegressionGP  ShowOutputSD=off  ShowOutputIntervals=off  Alpha=0.05  OutMin=[]  OutMax=[]  SDOutMin=[]  SDOutMax=[]  IntervalsOutMin=[]  IntervalsOutMax=[]  KernelMin=[]  KernelMax=[]  DistanceOutMin=[]  DistanceOutMax=[]  BasisOutMin=[]  BasisOutMax=[]  StandardizedInputOutMin=[]  StandardizedInputOutMax=[]  KernelParam1Min=[]  KernelParam1Max=[]  KernelParam2Min=[]  KernelParam2Max=[]  KernelParam3Min=[]  KernelParam3Max=[]  KernelParam4Min=[]  KernelParam4Max=[]  BasisParam1Min=[]  BasisParam1Max=[]  BasisParam2Min=[]  BasisParam2Max=[]  SDParam1Min=[]  SDParam1Max=[]  KernelParam5Min=[]  KernelParam5Max=[]
  Qp [m3/h] : Display  Commented=on
  Qp*Cp : Product
  R : Display  Commented=on
  Sum : Sum  Inputs=+-
  add2 : Sum  Inputs=+-
  di2 : Product  Inputs=/*
  Qc : Outport
  Pc : Outport  Port=2
  Cc : Outport  Port=3
  Qp : Outport  Port=4
  Cp : Outport  Port=5
  R [%] : Outport  Port=6
  wires:
  Cp RegressionNeuralNetwork Predict/1 -> Cp/1, [Cp], Cp [mg/L]/1
  Pc RegressionNeuralNetwork Predict/1 -> Pc/1, Pc [bar]/1
  Divide/1 -> 100%/1  "Recovery ratio (R)"
  Cf [mg/L]/1 -> Mux/3, [Cf]
  Mux/1 -> Pc RegressionNeuralNetwork Predict/1, Qp RegressionGP Predict/1, Cp RegressionNeuralNetwork Predict/1
  Pf [bar]/1 -> Mux/2
  Qf [m3/h]/1 -> [Qf], Qf [m3/h]1/1, Mux/1
  100%/1 -> R/1, R [%]/1
  Qp RegressionGP Predict/1 -> Qp/1, [Qp], Qp [m3/h]/1
  Sum/1 -> di2/1, Qc/1, Qc [m3/h]/1
  [Qf] -> Qf*Cf/1
  Qf*Cf/1 -> add2/1
  [Qp] -> Qp*Cp/1
  [Cf] -> Qf*Cf/2
  [Cp] -> Qp*Cp/2
  Qp*Cp/1 -> add2/2
  [Qf] -> Divide/1
  [Qp] -> Divide/2
  [Qf] -> Sum/1
  [Qp] -> Sum/2
  add2/1 -> di2/2
  di2/1 -> Cc/1, Cc [mg/L]/1

== system Sim_main/RO/PV2/RO num 6 ==
  note: Brine concentrate (Cc)
      | $C_c=(Q_f*C_f-Q_P*C_p)/Q_c$
  note: Concentrate flow rate (Qc)
      | $Qc=Qf-Qp$
  note: Recovery ratio (R)
      | $R=Q_p/Q_f$
  Qf [m3/h] : Inport
  Pf [bar] : Inport  Port=2
  Cf [mg/L] : Inport  Port=3
  100% : Gain  Gain=100
  Cc [mg/L] : Display  Commented=on
      settings: Format=bank
  Cp RegressionNeuralNetwork Predict : statsLibrary/Regression/RegressionNeuralNetwork Predict  TrainedLearner=RO_Cp.RegressionNeuralNetwork  OutMin=[]  OutMax=[]  OutputLayerOutMin=[]  OutputLayerOutMax=[]  OutputLayerAdditionOutMin=[]  OutputLayerAdditionOutMax=[]  LayerSelector=Layer 1  Layer1OutMin=[]  Layer1OutMax=[]  Layer1AdditionOutMin=[]  Layer1AdditionOutMax=[]  Layer2OutMin=[]  Layer2OutMax=[]  Layer2AdditionOutMin=[]  Layer2AdditionOutMax=[]  Layer3OutMin=[]  Layer3OutMax=[]  Layer3AdditionOutMin=[]  Layer3AdditionOutMax=[]  Layer4OutMin=[]  Layer4OutMax=[]  Layer4AdditionOutMin=[]  Layer4AdditionOutMax=[]  Layer5OutMin=[]  Layer5OutMax=[]  Layer5AdditionOutMin=[]  Layer5AdditionOutMax=[]  Layer6OutMin=[]  Layer6OutMax=[]  Layer6AdditionOutMin=[]  Layer6AdditionOutMax=[]  Layer7OutMin=[]  Layer7OutMax=[]  Layer7AdditionOutMin=[]  Layer7AdditionOutMax=[]  Layer8OutMin=[]  Layer8OutMax=[]  Layer8AdditionOutMin=[]  Layer8AdditionOutMax=[]  Layer9OutMin=[]  Layer9OutMax=[]  Layer9AdditionOutMin=[]  Layer9AdditionOutMax=[]  Layer10OutMin=[]  Layer10OutMax=[]  Layer10AdditionOutMin=[]  Layer10AdditionOutMax=[]  Layer11OutMin=[]  Layer11OutMax=[]  Layer11AdditionOutMin=[]  Layer11AdditionOutMax=[]  StandardizedInputOutMin=[]  StandardizedInputOutMax=[]  NumHiddenLayers=1
  Cp [mg/L] : Display  Commented=on
  Divide : Product  Inputs=/*
  Mux : Mux  Inputs=3
  Pc RegressionNeuralNetwork Predict : statsLibrary/Regression/RegressionNeuralNetwork Predict  TrainedLearner=RO_Pc.RegressionNeuralNetwork  OutMin=[]  OutMax=[]  OutputLayerOutMin=[]  OutputLayerOutMax=[]  OutputLayerAdditionOutMin=[]  OutputLayerAdditionOutMax=[]  LayerSelector=Layer 1  Layer1OutMin=[]  Layer1OutMax=[]  Layer1AdditionOutMin=[]  Layer1AdditionOutMax=[]  Layer2OutMin=[]  Layer2OutMax=[]  Layer2AdditionOutMin=[]  Layer2AdditionOutMax=[]  Layer3OutMin=[]  Layer3OutMax=[]  Layer3AdditionOutMin=[]  Layer3AdditionOutMax=[]  Layer4OutMin=[]  Layer4OutMax=[]  Layer4AdditionOutMin=[]  Layer4AdditionOutMax=[]  Layer5OutMin=[]  Layer5OutMax=[]  Layer5AdditionOutMin=[]  Layer5AdditionOutMax=[]  Layer6OutMin=[]  Layer6OutMax=[]  Layer6AdditionOutMin=[]  Layer6AdditionOutMax=[]  Layer7OutMin=[]  Layer7OutMax=[]  Layer7AdditionOutMin=[]  Layer7AdditionOutMax=[]  Layer8OutMin=[]  Layer8OutMax=[]  Layer8AdditionOutMin=[]  Layer8AdditionOutMax=[]  Layer9OutMin=[]  Layer9OutMax=[]  Layer9AdditionOutMin=[]  Layer9AdditionOutMax=[]  Layer10OutMin=[]  Layer10OutMax=[]  Layer10AdditionOutMin=[]  Layer10AdditionOutMax=[]  Layer11OutMin=[]  Layer11OutMax=[]  Layer11AdditionOutMin=[]  Layer11AdditionOutMax=[]  StandardizedInputOutMin=[]  StandardizedInputOutMax=[]  NumHiddenLayers=1
  Pc [bar] : Display  Commented=on
  Qc [m3/h] : Display  Commented=on
  Qf*Cf : Product
  Qp RegressionGP Predict : statsLibrary/Regression/RegressionGP Predict  TrainedLearner=RO_Qp.RegressionGP  ShowOutputSD=off  ShowOutputIntervals=off  Alpha=0.05  OutMin=[]  OutMax=[]  SDOutMin=[]  SDOutMax=[]  IntervalsOutMin=[]  IntervalsOutMax=[]  KernelMin=[]  KernelMax=[]  DistanceOutMin=[]  DistanceOutMax=[]  BasisOutMin=[]  BasisOutMax=[]  StandardizedInputOutMin=[]  StandardizedInputOutMax=[]  KernelParam1Min=[]  KernelParam1Max=[]  KernelParam2Min=[]  KernelParam2Max=[]  KernelParam3Min=[]  KernelParam3Max=[]  KernelParam4Min=[]  KernelParam4Max=[]  BasisParam1Min=[]  BasisParam1Max=[]  BasisParam2Min=[]  BasisParam2Max=[]  SDParam1Min=[]  SDParam1Max=[]  KernelParam5Min=[]  KernelParam5Max=[]
  Qp [m3/h] : Display  Commented=on
  Qp*Cp : Product
  R : Display  Commented=on
  Sum : Sum  Inputs=+-
  add2 : Sum  Inputs=+-
  di2 : Product  Inputs=/*
  Qc : Outport
  Pc : Outport  Port=2
  Cc : Outport  Port=3
  Qp : Outport  Port=4
  Cp : Outport  Port=5
  R [%] : Outport  Port=6
  wires:
  di2/1 -> Cc [mg/L]/1, Cc/1
  add2/1 -> di2/2
  [Qp] -> Sum/2
  [Qf] -> Sum/1
  [Qp] -> Divide/2
  [Qf] -> Divide/1
  Qp*Cp/1 -> add2/2
  [Cp] -> Qp*Cp/2
  [Cf] -> Qf*Cf/2
  [Qp] -> Qp*Cp/1
  Qf*Cf/1 -> add2/1
  [Qf] -> Qf*Cf/1
  Sum/1 -> Qc [m3/h]/1, Qc/1, di2/1
  Qp RegressionGP Predict/1 -> Qp [m3/h]/1, [Qp], Qp/1
  100%/1 -> R [%]/1, R/1
  Qf [m3/h]/1 -> Mux/1, [Qf]
  Pf [bar]/1 -> Mux/2
  Mux/1 -> Cp RegressionNeuralNetwork Predict/1, Qp RegressionGP Predict/1, Pc RegressionNeuralNetwork Predict/1
  Cf [mg/L]/1 -> [Cf], Mux/3
  Divide/1 -> 100%/1  "Recovery ratio (R)"
  Pc RegressionNeuralNetwork Predict/1 -> Pc [bar]/1, Pc/1
  Cp RegressionNeuralNetwork Predict/1 -> Cp [mg/L]/1, [Cp], Cp/1

== system Sim_main/RO/PV2/Subsystem ==
  note: product concentrate (Cp)
      | $C_3=(Q_1*C_1+Q_2*C_2)/Q_3$
  In1 : Inport
  In2 : Inport  Port=2
  In3 : Inport  Port=3
  In4 : Inport  Port=4
  Add1 : Sum
  Q1*C1 : Product
  Q2*C2 : Product
  add2 : Sum
  di2 : Product  Inputs=/*
  Out1 : Outport
  Out2 : Outport  Port=2
  wires:
  add2/1 -> di2/2
  In1/1 -> Add1/1, Q1*C1/1
  di2/1 -> Out1/1
  In3/1 -> Add1/2, Q2*C2/1
  Q1*C1/1 -> add2/1
  Q2*C2/1 -> add2/2
  Add1/1 -> di2/1, Out2/1
  In2/1 -> Q1*C1/2
  In4/1 -> Q2*C2/2

== system Sim_main/RO/PV2/Subsystem1 ==
  note: product concentrate (Cp)
      | $C_3=(Q_1*C_1+Q_2*C_2)/Q_3$
  In2 : Inport
  In3 : Inport  Port=2
  In4 : Inport  Port=3
  In1 : Inport  Port=4
  Add2 : Sum
  Q1*C1 : Product
  Q2*C2 : Product
  add2 : Sum
  di2 : Product  Inputs=/*
  Out1 : Outport
  Out2 : Outport  Port=2
  wires:
  di2/1 -> Out1/1
  add2/1 -> di2/2
  Q1*C1/1 -> add2/1
  Add2/1 -> di2/1, Out2/1
  In3/1 -> Q2*C2/1, Add2/2
  In4/1 -> Q2*C2/2
  Q2*C2/1 -> add2/2
  In2/1 -> Add2/1, Q1*C1/2
  In1/1 -> Q1*C1/1

== system Sim_main/RO/PV2/Subsystem2 ==
  note: product concentrate (Cp)
      | $C_3=(Q_1*C_1+Q_2*C_2)/Q_3$
  In2 : Inport
  In3 : Inport  Port=2
  In4 : Inport  Port=3
  In1 : Inport  Port=4
  Add2 : Sum
  Q1*C1 : Product
  Q2*C2 : Product
  add2 : Sum
  di2 : Product  Inputs=/*
  Out1 : Outport
  Out2 : Outport  Port=2
  wires:
  In1/1 -> Q1*C1/1
  In2/1 -> Q1*C1/2, Add2/1
  Q2*C2/1 -> add2/2
  In4/1 -> Q2*C2/2
  In3/1 -> Add2/2, Q2*C2/1
  Add2/1 -> Out2/1, di2/1
  Q1*C1/1 -> add2/1
  add2/1 -> di2/2
  di2/1 -> Out1/1

== system Sim_main/RO/PV2/Subsystem3 ==
  note: product concentrate (Cp)
      | $C_3=(Q_1*C_1+Q_2*C_2)/Q_3$
  In2 : Inport
  In3 : Inport  Port=2
  In4 : Inport  Port=3
  In1 : Inport  Port=4
  Add2 : Sum
  Q1*C1 : Product
  Q2*C2 : Product
  add2 : Sum
  di2 : Product  Inputs=/*
  Out1 : Outport
  wires:
  di2/1 -> Out1/1
  add2/1 -> di2/2
  Q1*C1/1 -> add2/1
  Add2/1 -> di2/1
  In3/1 -> Q2*C2/1, Add2/2
  In4/1 -> Q2*C2/2
  Q2*C2/1 -> add2/2
  In2/1 -> Add2/1, Q1*C1/2
  In1/1 -> Q1*C1/1

== system Sim_main/RO/PV2/Subsystem5 ==
  note: product concentrate (Cp)
      | $C_3=(Q_1*C_1+Q_2*C_2)/Q_3$
  In2 : Inport
  In3 : Inport  Port=2
  In4 : Inport  Port=3
  In1 : Inport  Port=4
  Add2 : Sum
  Q1*C1 : Product
  Q2*C2 : Product
  add2 : Sum
  di2 : Product  Inputs=/*
  Out1 : Outport
  Out2 : Outport  Port=2
  wires:
  In1/1 -> Q1*C1/1
  In2/1 -> Q1*C1/2, Add2/1
  Q2*C2/1 -> add2/2
  In4/1 -> Q2*C2/2
  In3/1 -> Add2/2, Q2*C2/1
  Add2/1 -> Out2/1, di2/1
  Q1*C1/1 -> add2/1
  add2/1 -> di2/2
  di2/1 -> Out1/1

== matlab function Sim_main/Compressor and Air tank/MATLAB Function ==
  settings: updateMethod=DISCRETE
  data: currentLevel input; valveState output; maxLevel input; minLevel input
function valveState = valveControl(currentLevel, maxLevel, minLevel)
    % Initialize persistent variable to store previous state
    persistent prevState;
    if isempty(prevState)
        prevState = 0; % Start with valve closed
    end

    % Valve Control Logic
    if currentLevel >= maxLevel && prevState == 0
        valveState = 1; % Open valve
    elseif currentLevel <= minLevel && prevState == 1
        valveState = 0; % Close valve
    else
        valveState = prevState; % Maintain previous state (hysteresis)
    end

    prevState = valveState; % Store current state for next call
end
